simulink model "effec_wn_naturalfrequencet"  (R2023b)
settings: Solver=VariableStepAuto  StartTime=0.0  StopTime=10.0  RelTol=1e-3
settings Model: Creator=hp  LastModifiedBy=hp

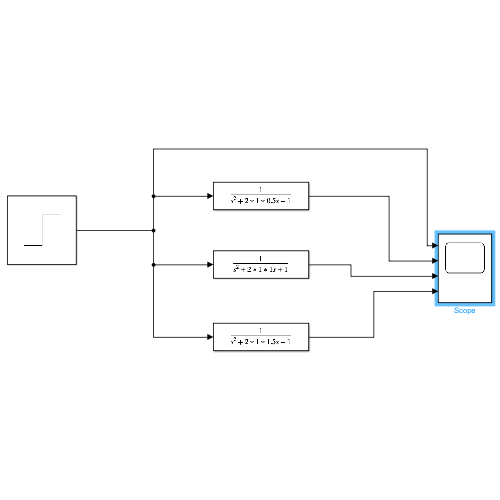
[thumbnail: Simulink's stored preview of the top-level diagram]
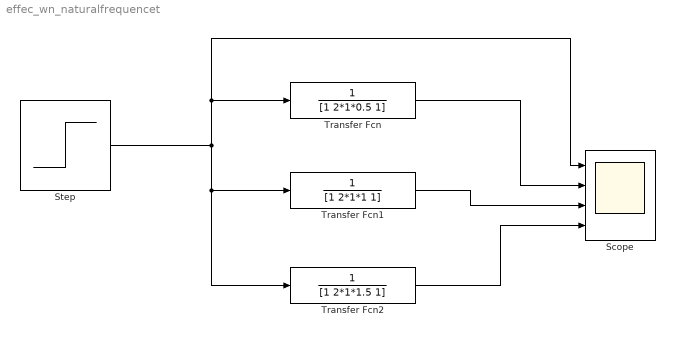
== system effec_wn_naturalfrequencet ==
  Scope : Scope  NumInputPorts=4
  Step : Step  SampleTime=0
  Transfer Fcn : TransferFcn  Denominator=[1 2*1*0.5 1]
  Transfer Fcn1 : TransferFcn  Denominator=[1 2*1*1 1]
  Transfer Fcn2 : TransferFcn  Denominator=[1 2*1*1.5 1]
  wires:
  Step/1 -> Scope/1, Transfer Fcn/1, Transfer Fcn2/1, Transfer Fcn1/1
  Transfer Fcn1/1 -> Scope/3
  Transfer Fcn/1 -> Scope/2
  Transfer Fcn2/1 -> Scope/4
